simulink model "Model_P0"  (R2022b)
settings: Solver=FixedStepAuto  StartTime=0.0  StopTime=10000  FixedStep=1  RelTol=1e-3
undefined symbols (not defined in the file): epsilon, OCV, OCV_Delta, R0, SOC_levels
settings Model: Creator=frederikvanmaele  LastModifiedBy=AdministratorDevice
settings DebuggingCC: UnconnectedInputMsg=warning  UnconnectedOutputMsg=warning  UnconnectedLineMsg=warning
settings ModelReferenceCC: EnableRefExpFcnMdlSchedulingChecks=on
settings RTWCC: DLArmComputeVersion=19.05

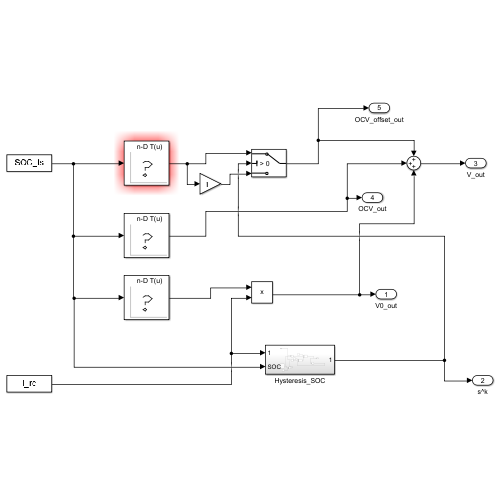
[thumbnail: Simulink's stored preview of the top-level diagram]
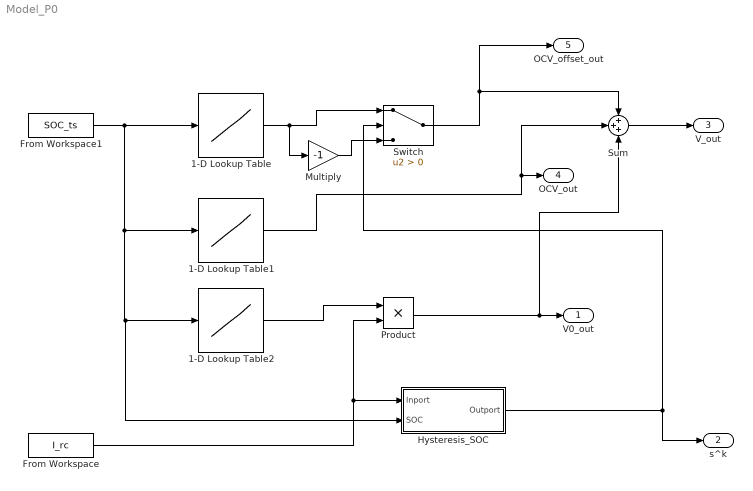
== system Model_P0 ==
  1-D Lookup Table : Lookup_n-D  NumberOfTableDimensions=1  BreakpointsForDimension1=SOC_levels  Table=OCV_Delta  InternalRulePriority=Speed  RndMeth=Simplest
  1-D Lookup Table1 : Lookup_n-D  NumberOfTableDimensions=1  BreakpointsForDimension1=SOC_levels  Table=OCV  InternalRulePriority=Speed  RndMeth=Simplest
  1-D Lookup Table2 : Lookup_n-D  NumberOfTableDimensions=1  BreakpointsForDimension1=SOC_levels  Table=R0  InternalRulePriority=Speed  RndMeth=Simplest
  From Workspace : FromWorkspace  VariableName=I_rc
  From Workspace1 : FromWorkspace  VariableName=SOC_ts
  Hysteresis_SOC : Subsystem
  Multiply : Gain  Gain=-1
  Product : Product
  Sum : Sum  Inputs=+++
  Switch : Switch  Criteria=u2 > Threshold  SaturateOnIntegerOverflow=off  InputSameDT=off
  V0_out : Outport
  s^k : Outport  Port=2
  V_out : Outport  Port=3
  OCV_out : Outport  Port=4
  OCV_offset_out : Outport  Port=5
  wires:
  From Workspace/1 -> Product/2, Hysteresis_SOC/1(Inport)
  Product/1 -> V0_out/1, Sum/3
  Hysteresis_SOC/1(Outport) -> s^k/1, Switch/2
  1-D Lookup Table/1 -> Multiply/1, Switch/1
  Multiply/1 -> Switch/3
  Switch/1 -> OCV_offset_out/1, Sum/1
  1-D Lookup Table1/1 -> OCV_out/1, Sum/2
  Sum/1 -> V_out/1
  From Workspace1/1 -> Hysteresis_SOC/2(SOC), 1-D Lookup Table2/1, 1-D Lookup Table1/1, 1-D Lookup Table/1
  1-D Lookup Table2/1 -> Product/1

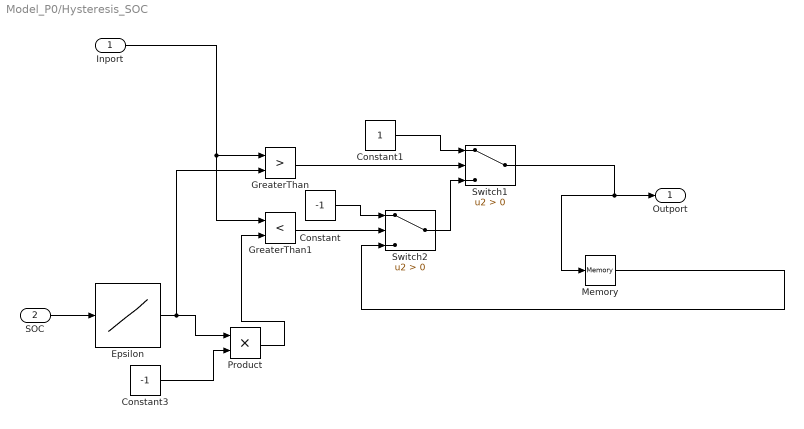
== system Model_P0/Hysteresis_SOC ==
  Inport : Inport
  SOC : Inport  Port=2
  Constant : Constant  Value=-1
  Constant1 : Constant
  Constant3 : Constant  Value=-1
  Epsilon : Lookup_n-D  NumberOfTableDimensions=1  BreakpointsForDimension1=SOC_levels  Table=epsilon  InternalRulePriority=Speed  RndMeth=Simplest
  GreaterThan : RelationalOperator  Operator=>  OutDataTypeStr=boolean  RndMeth=Simplest  InputSameDT=off
  GreaterThan1 : RelationalOperator  Operator=<  OutDataTypeStr=boolean  RndMeth=Simplest  InputSameDT=off
  Memory : Memory
  Product : Product
  Switch1 : Switch  Criteria=u2 > Threshold  SaturateOnIntegerOverflow=off  InputSameDT=off
  Switch2 : Switch  Criteria=u2 > Threshold  SaturateOnIntegerOverflow=off  InputSameDT=off
  Outport : Outport
  wires:
  GreaterThan1/1 -> Switch2/2
  Constant/1 -> Switch2/1
  Switch1/1 -> Outport/1, Memory/1
  Inport/1 -> GreaterThan1/1, GreaterThan/1
  Constant1/1 -> Switch1/1
  Switch2/1 -> Switch1/3
  GreaterThan/1 -> Switch1/2
  Memory/1 -> Switch2/3
  SOC/1 -> Epsilon/1
  Epsilon/1 -> GreaterThan/2, Product/1
  Constant3/1 -> Product/2
  Product/1 -> GreaterThan1/2
